simulink subsystem "subrQuadRotation"  (R2024a)
settings: Solver=VariableStepAuto  StartTime=0.0  StopTime=10.0  RelTol=1e-3
model mask{TorqueMap=[1,1,1,1], MomentArm=[0,0,0,0], RotJ=1, RotB=0, PosnIC=0, RateIC=0}
  mask prompts: TorqueMap "Torque Map"; MomentArm "Moment Arm"; RotJ "Moment of Inertia"; RotB "Aero Viscous Friction"; PosnIC "Position IC"; RateIC "Rate IC"
undefined symbols (not defined in the file): AeroB
settings Model: Creator=anant  LastModifiedBy=anant

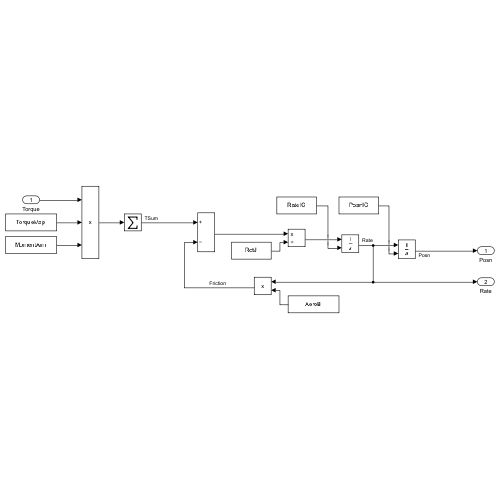
[thumbnail: Simulink's stored preview of the top-level diagram]
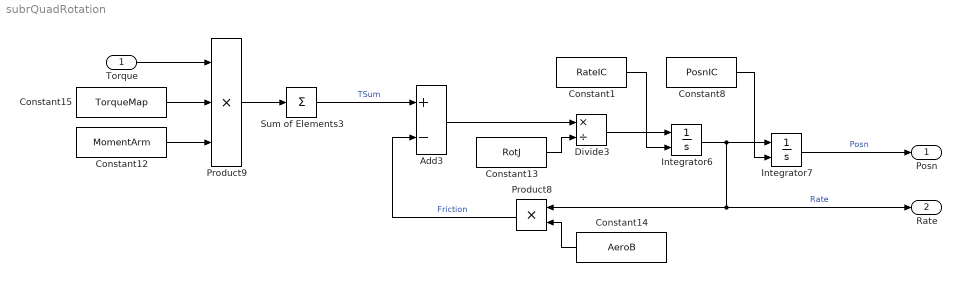
== system subrQuadRotation ==
  Torque : Inport
  Add3 : Sum  Inputs=+-
  Constant1 : Constant  Value=RateIC
  Constant12 : Constant  Value=MomentArm
  Constant13 : Constant  Value=RotJ
  Constant14 : Constant  Value=AeroB
  Constant15 : Constant  Value=TorqueMap
  Constant8 : Constant  Value=PosnIC
  Divide3 : Product  Inputs=*/
  Integrator6 : Integrator  InitialConditionSource=external
  Integrator7 : Integrator  InitialConditionSource=external
  Product8 : Product
  Product9 : Product  Inputs=3
  Sum of Elements3 : Sum  Inputs=+
  Posn : Outport
  Rate : Outport  Port=2
  wires:
  Constant15/1 -> Product9/2
  Product8/1 -> Add3/2  "Friction"
  Integrator6/1 -> Product8/1, Rate/1, Integrator7/1  "Rate"
  Product9/1 -> Sum of Elements3/1
  Constant12/1 -> Product9/3
  Constant13/1 -> Divide3/2
  Constant8/1 -> Integrator7/2
  Add3/1 -> Divide3/1
  Sum of Elements3/1 -> Add3/1  "TSum"
  Constant14/1 -> Product8/2
  Divide3/1 -> Integrator6/1
  Torque/1 -> Product9/1
  Integrator7/1 -> Posn/1  "Posn"
  Constant1/1 -> Integrator6/2
